simulink model "StraightLine"  (R2015b)
settings: Solver=VariableStepAuto  StartTime=0.0  StopTime=2000  RelTol=1e-3
values from neighbouring files (symbols this model uses):
  aa = a(i)    [BeardMethod.m]
  alpha = 1.65    [BeardMethod.m]    (also in OrbitCenter.m = abs((ang1-ang2)/2); RevisedMethod.m)
  ang = angle(i)    [BeardMethod.m]    (also in RevisedMethod.m = 0)
  bb = b(i)    [BeardMethod.m]
  chi_inf = pi/2    (= 1.57079632679)    [BeardMethod.m]    (also in RevisedMethod.m)
  course_int = course_int+2*pi    (= 6.28318530718)    [BeardMethod.m]    (also in RevisedMethod.m = -0.785398163397)
  endx = E2(1)-6    [BeardMethod.m]    (also in RevisedMethod.m = 300)
  epsi = 0.1    [BeardMethod.m]    (also in RevisedMethod.m = 0.5)
  i = 1    [BeardMethod.m]    (also in RevisedMethod.m = 1, go left, x decreases))
  k = 0.02    [BeardMethod.m]    (also in RevisedMethod.m = 0.1)
  kk = pi/2    (= 1.57079632679)    [BeardMethod.m]    (also in RevisedMethod.m)
  phiw = 230/180*pi    (= 4.01425727959)    [BeardMethod.m]    (also in RevisedMethod.m)
  Va = 13    [BeardMethod.m]    (also in RevisedMethod.m)
  w = 0.9    [BeardMethod.m]
  x_int = x.data(end)    [BeardMethod.m]    (also in RevisedMethod.m = 0)
  y_int = y.data(end)    [BeardMethod.m]    (also in RevisedMethod.m = 80)
libraries: simulink x1
settings Model: Creator=Bingyu Zhou  LastModifiedBy=Bingyu Zhou

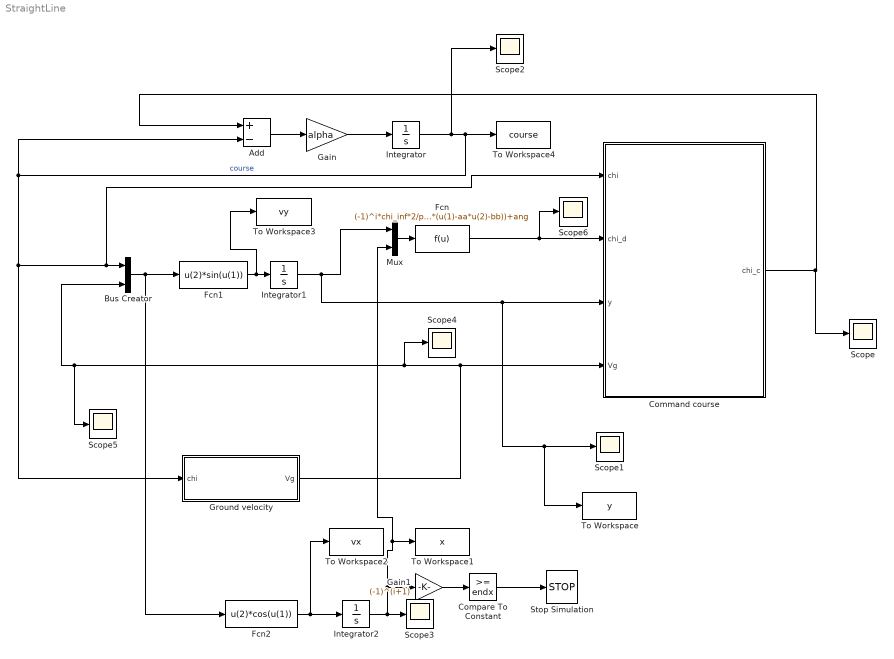
== system StraightLine ==
  Add : Sum  Inputs=+-
  Bus Creator : BusCreator  Inputs=2
  Command course : Subsystem
  Compare To Constant : simulink/Logic and Bit Operations/Compare To Constant  relop=>=  const=endx  OutDataTypeStr=boolean
  Fcn : Fcn  Expr=(-1)^i*chi_inf*2/pi*atan(k*(u(1)-aa*u(2)-bb))+ang
  Fcn1 : Fcn  Expr=u(2)*sin(u(1))
  Fcn2 : Fcn  Expr=u(2)*cos(u(1))
  Gain : Gain  Gain=alpha
  Gain1 : Gain  Gain=(-1)^(i+1)
  Ground velocity : Subsystem
  Integrator : Integrator  InitialCondition=course_int
  Integrator1 : Integrator  InitialCondition=y_int
  Integrator2 : Integrator  InitialCondition=x_int
  Mux : Mux  Inputs=2
  Scope{,1..6} (7 alike) : Scope
  Stop Simulation : Stop
  To Workspace : ToWorkspace  VariableName=y  SaveFormat=Timeseries  SampleTime=-1
  To Workspace1 : ToWorkspace  VariableName=x  SaveFormat=Timeseries  SampleTime=-1
  To Workspace2 : ToWorkspace  VariableName=vx  SaveFormat=Timeseries  SampleTime=-1
  To Workspace3 : ToWorkspace  VariableName=vy  SaveFormat=Timeseries  SampleTime=-1
  To Workspace4 : ToWorkspace  VariableName=course  SaveFormat=Timeseries  SampleTime=-1
  wires:
  Add/1 -> Gain/1
  Gain/1 -> Integrator/1
  Integrator/1 -> Scope2/1, To Workspace4/1, Add/2, Command course/1(chi), Bus Creator/1, Ground velocity/1(chi)  "course"
  Bus Creator/1 -> Fcn2/1, Fcn1/1
  Fcn1/1 -> To Workspace3/1, Integrator1/1
  Integrator1/1 -> Mux/1, Command course/3(y), To Workspace/1, Scope1/1
  Fcn/1 -> Scope6/1, Command course/2(chi_d)
  Command course/1(chi_c) -> Scope/1, Add/1
  Fcn2/1 -> To Workspace2/1, Integrator2/1
  Integrator2/1 -> Gain1/1, Mux/2, To Workspace1/1, Scope3/1
  Ground velocity/1(Vg) -> Scope5/1, Bus Creator/2, Scope4/1, Command course/4(Vg)
  Mux/1 -> Fcn/1
  Compare To Constant/1 -> Stop Simulation/1
  Gain1/1 -> Compare To Constant/1

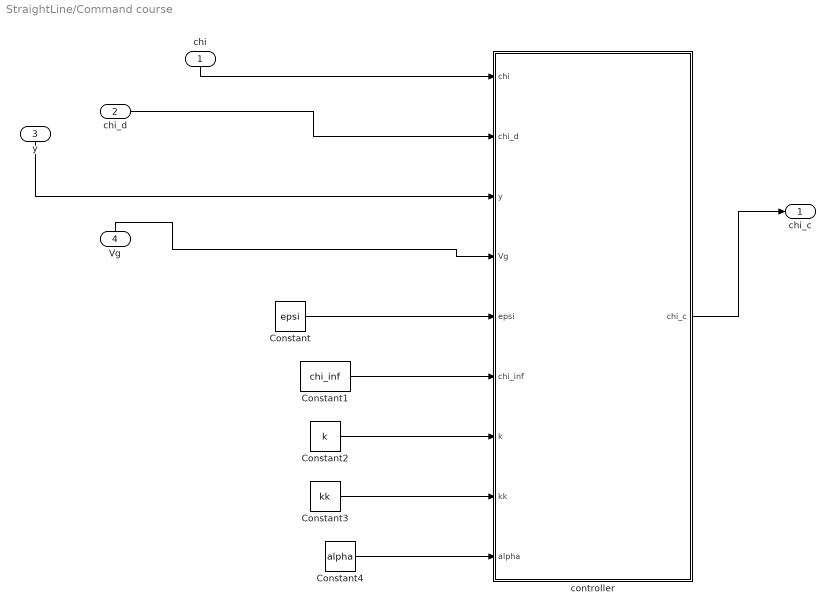
== system StraightLine/Command course ==
  chi : Inport
  chi_d : Inport  Port=2
  y : Inport  Port=3
  Vg : Inport  Port=4
  Constant : Constant  Value=epsi
  Constant1 : Constant  Value=chi_inf
  Constant2 : Constant  Value=k
  Constant3 : Constant  Value=kk
  Constant4 : Constant  Value=alpha
  controller : MATLAB Function  TreatAsAtomicUnit=on
  chi_c : Outport
  wires:
  chi_d/1 -> controller/2(chi_d)
  controller/1(chi_c) -> chi_c/1
  chi/1 -> controller/1(chi)
  Vg/1 -> controller/4(Vg)
  Constant1/1 -> controller/6(chi_inf)
  Constant/1 -> controller/5(epsi)
  Constant2/1 -> controller/7(k)
  Constant3/1 -> controller/8(kk)
  y/1 -> controller/3(y)
  Constant4/1 -> controller/9(alpha)

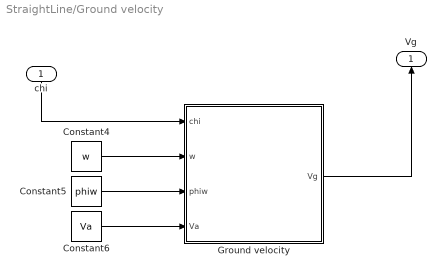
== system StraightLine/Ground velocity ==
  chi : Inport
  Constant4 : Constant  Value=w
  Constant5 : Constant  Value=phiw
  Constant6 : Constant  Value=Va
  Ground velocity : MATLAB Function  TreatAsAtomicUnit=on
  Vg : Outport
  wires:
  Ground velocity/1(Vg) -> Vg/1
  chi/1 -> Ground velocity/1(chi)
  Constant6/1 -> Ground velocity/4(Va)
  Constant5/1 -> Ground velocity/3(phiw)
  Constant4/1 -> Ground velocity/2(w)

== matlab function StraightLine/Ground velocity/Ground velocity ==
  data: chi input; Vg output; w input; phiw input; Va input
function Vg = GroundVelocity(chi,w,phiw,Va)
%generate the ground velocity based on course angle
Vg=w*cos(chi-phiw)+sqrt(Va^2-w^2*(sin(chi-phiw))^2);
end

== matlab function StraightLine/Command course/controller ==
  data: chi input; chi_d input; y input; Vg input; chi_c output; epsi input; chi_inf input; k input; kk input; alpha input
function chi_c = CommandCourse(chi,chi_d,y,Vg,epsi,chi_inf,k,kk,alpha)
%generate command course angle chi_c
sat=(chi-chi_d)/epsi;
if abs(sat)<=1
    rho=sat;
else
    rho=sign(sat);
end
chi_c=chi-chi_inf*2/pi/alpha*k/(1+(k*y)^2)*Vg*sin(chi)-kk/alpha*rho;


end
